simulink model "T1"  (R2024a)
settings: Solver=VariableStepAuto  StartTime=0.0  StopTime=6  RelTol=1e-3
libraries: cstblocks x2
settings Model: Creator=PMYLS  LastModifiedBy=PMYLS

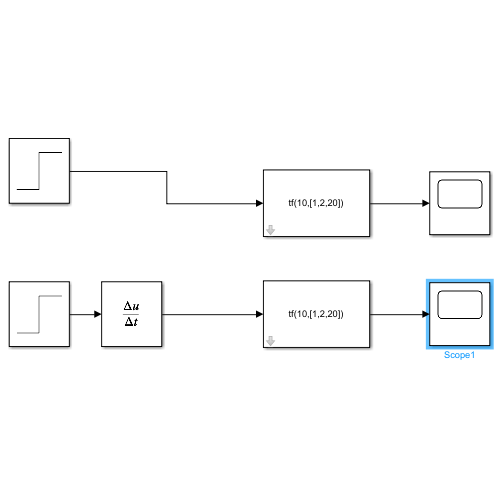
[thumbnail: Simulink's stored preview of the top-level diagram]
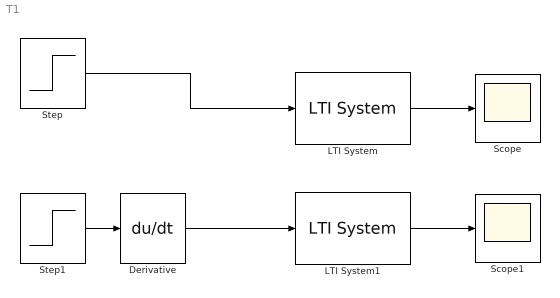
== system T1 ==
  Derivative : Derivative
  LTI System : cstblocks/LTI System  sys=tf(10,[1,2,20])  IC=[]  PadeOrder=0
  LTI System1 : cstblocks/LTI System  sys=tf(10,[1,2,20])  IC=[]  PadeOrder=0
  Scope : Scope
  Scope1 : Scope
  Step : Step  SampleTime=0
  Step1 : Step  SampleTime=0
  wires:
  LTI System/1 -> Scope/1
  Step1/1 -> Derivative/1
  Step/1 -> LTI System/1
  LTI System1/1 -> Scope1/1
  Derivative/1 -> LTI System1/1
